simulink model "tutorial_simulink_4"  (R2024b)
settings: Solver=VariableStepAuto  StartTime=0.0  StopTime=10.0  RelTol=1e-3
settings Model: Creator=俞书阳  LastModifiedBy=user

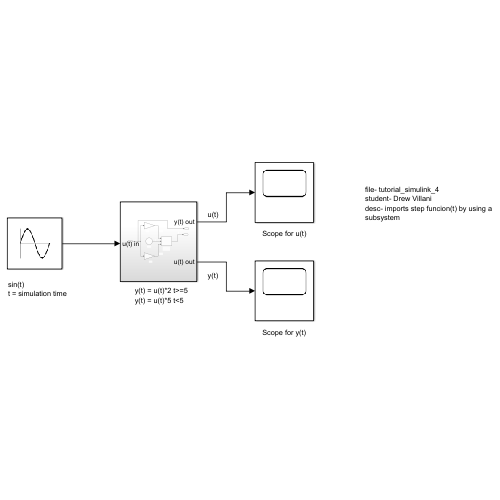
[thumbnail: Simulink's stored preview of the top-level diagram]
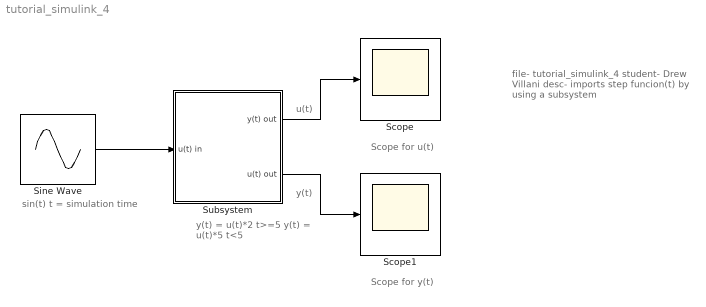
== system tutorial_simulink_4 ==
  note: sin(t)
      | t = simulation time
  note: y(t) = u(t)*2 t>=5
      | y(t) = u(t)*5 t<5
  note: u(t)
  note: file- tutorial_simulink_4
      | student- Drew Villani
      | desc- imports step funcion(t) by using a
      | subsystem
  note: Scope for u(t)
  note: y(t)
  note: Scope for y(t)
  Scope : Scope
  Scope1 : Scope
  Sine Wave : Sin  SampleTime=0
  Subsystem : Subsystem
  wires:
  Sine Wave/1 -> Subsystem/1(u(t) in)
  Subsystem/1(y(t) out) -> Scope/1
  Subsystem/2(u(t) out) -> Scope1/1

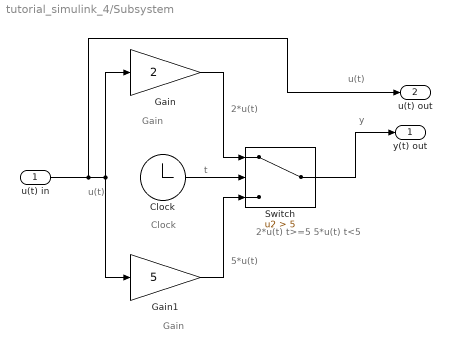
== system tutorial_simulink_4/Subsystem ==
  note: u(t)
  note: y
  note: 2*u(t) t>=5
      | 5*u(t) t<5
  note: 5*u(t)
  note: 2*u(t)
  note: Gain
  note: Gain
  note: t
  note: Clock
  note: u(t)
  u(t) in : Inport
  Clock : Clock
  Gain : Gain  Gain=2
  Gain1 : Gain  Gain=5
  Switch : Switch  Criteria=u2 > Threshold  Threshold=5  SaturateOnIntegerOverflow=off  InputSameDT=off
  y(t) out : Outport
  u(t) out : Outport  Port=2
  wires:
  Switch/1 -> y(t) out/1
  Gain1/1 -> Switch/3
  Gain/1 -> Switch/1
  Clock/1 -> Switch/2
  u(t) in/1 -> u(t) out/1, Gain1/1, Gain/1
